simulink model "discretization_example_student"  (R2022b)
settings: Solver=ode4  StartTime=0.0  StopTime=timeEnd  FixedStep=timeStep  RelTol=1e-3
values from neighbouring files (symbols this model uses):
  stateInit = [1; 0.5]    [discretization_example_init.m]
  timeStep = 1e-3    (= 0.001)    [discretization_example_init.m]
undefined symbols (not defined in the file or in its folder): sys
settings Model: Creator=maam  LastModifiedBy=15043
settings SolverCC: AlgebraicLoopSolver=TrustRegion
settings DebuggingCC: UnconnectedInputMsg=warning  UnconnectedOutputMsg=warning  UnconnectedLineMsg=warning  SFMachineParentedDataDiag=warning  ArithmeticOperatorsInVariantConditions=warning
settings ModelReferenceCC: EnableRefExpFcnMdlSchedulingChecks=on
settings SFSimCC: CustomCodeUndefinedFunction=UseInterfaceOnly
settings CodeAppCC: StateflowObjectComments=on

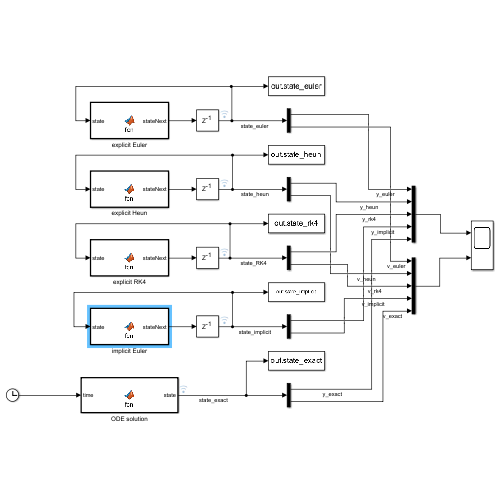
[thumbnail: Simulink's stored preview of the top-level diagram]
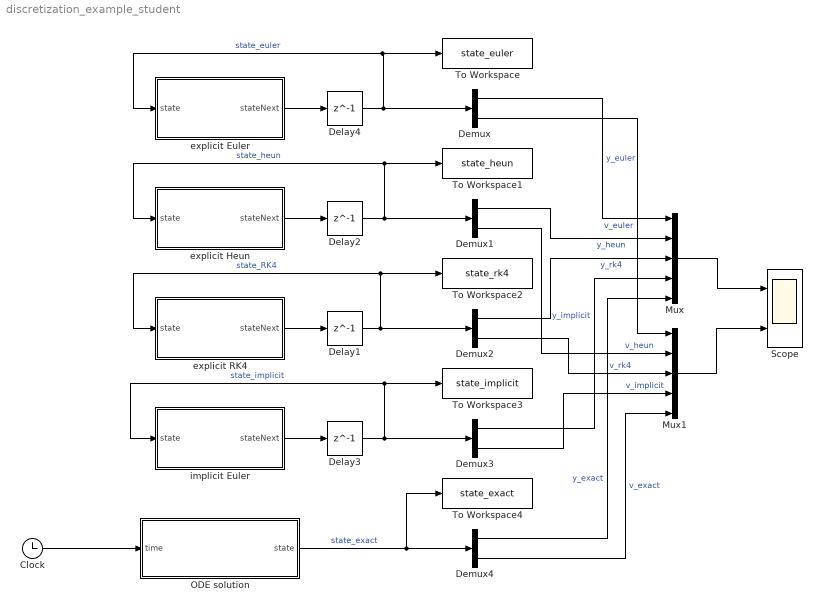
== system discretization_example_student ==
  Clock : Clock
  Delay{1..4} (4 alike) : Delay  DelayLength=1  InitialCondition=stateInit
  Demux{,1..4} (5 alike) : Demux  Outputs=2
  Mux : Mux  Inputs=5
  Mux1 : Mux  Inputs=5
  ODE solution : MATLAB Function  TreatAsAtomicUnit=on
  Scope : Scope  NumInputPorts=2
  To Workspace : ToWorkspace  VariableName=state_euler  SaveFormat=Timeseries  SampleTime=-1
  To Workspace1 : ToWorkspace  VariableName=state_heun  SaveFormat=Timeseries  SampleTime=-1
  To Workspace2 : ToWorkspace  VariableName=state_rk4  SaveFormat=Timeseries  SampleTime=-1
  To Workspace3 : ToWorkspace  VariableName=state_implicit  SaveFormat=Timeseries  SampleTime=-1
  To Workspace4 : ToWorkspace  VariableName=state_exact  SaveFormat=Timeseries  SampleTime=-1
  explicit Euler : MATLAB Function  TreatAsAtomicUnit=on
  explicit Heun : MATLAB Function  TreatAsAtomicUnit=on
  explicit RK4 : MATLAB Function  TreatAsAtomicUnit=on
  implicit Euler : MATLAB Function  TreatAsAtomicUnit=on
  wires:
  explicit Euler/1(stateNext) -> Delay4/1
  implicit Euler/1(stateNext) -> Delay3/1
  Clock/1 -> ODE solution/1(time)
  ODE solution/1(state) -> Demux4/1, To Workspace4/1  "state_exact"
  explicit RK4/1(stateNext) -> Delay1/1
  explicit Heun/1(stateNext) -> Delay2/1
  Delay3/1 -> Demux3/1, implicit Euler/1(state), To Workspace3/1  "state_implicit"
  Delay1/1 -> Demux2/1, To Workspace2/1, explicit RK4/1(state)  "state_RK4"
  Delay2/1 -> Demux1/1, To Workspace1/1, explicit Heun/1(state)  "state_heun"
  Delay4/1 -> Demux/1, To Workspace/1, explicit Euler/1(state)  "state_euler"
  Mux1/1 -> Scope/2
  Mux/1 -> Scope/1
  Demux/1 -> Mux/1  "y_euler"
  Demux/2 -> Mux1/1  "v_euler"
  Demux1/1 -> Mux/2  "y_heun"
  Demux2/1 -> Mux/3  "y_rk4"
  Demux3/1 -> Mux/4  "y_implicit"
  Demux4/1 -> Mux/5  "y_exact"
  Demux1/2 -> Mux1/2  "v_heun"
  Demux2/2 -> Mux1/3  "v_rk4"
  Demux3/2 -> Mux1/4  "v_implicit"
  Demux4/2 -> Mux1/5  "v_exact"

== matlab function discretization_example_student/explicit Heun ==
  data: state input size=2; stateNext output size=2; timeStep parameter; sys parameter
function stateNext = fcn(state, timeStep, sys)

    h = timeStep;
    f = mass_spring_model_ode(0,state,sys);

    yNext = state + h * f;
    stateNext = state + h/2 * (f + mass_spring_model_ode(0+h,yNext,sys));


    function dy = mass_spring_model_ode(t, y, sys)
        % y(1) = p; y(2) = p_dot
        dy = zeros(2,1);
        dy(1) = y(2); 
        dy(2) = (-1/sys.mass)*(sys.damping*y(2) + sys.stiffness*y(1));
    end
end

== matlab function discretization_example_student/explicit Euler ==
  data: state input size=2; stateNext output size=2; timeStep parameter; sys parameter
function stateNext = fcn(state, timeStep, sys)

    h = timeStep;
    f = mass_spring_model_ode(0,state,sys);
    stateNext = state + h * f;
    
    function dy = mass_spring_model_ode(t, y, sys)
        % y(1) = p; y(2) = p_dot
        dy = zeros(2,1);
        dy(1) = y(2); 
        dy(2) = (-1/sys.mass)*(sys.damping*y(2) + sys.stiffness*y(1));
    end
end

== matlab function discretization_example_student/explicit RK4 ==
  data: state input size=2; stateNext output size=2; timeStep parameter; sys parameter
function stateNext = fcn(state, timeStep, sys)

    h = timeStep;
    s1 = mass_spring_model_ode(0,state,sys);
    s2 = mass_spring_model_ode(0+h/2,state+h/2*s1,sys);
    s3 = mass_spring_model_ode(0+h/2,state+h/2*s2,sys);
    s4 = mass_spring_model_ode(0+h,state+h*s3,sys);


    stateNext = state + h/6 * (s1+2*s2+2*s3+s4);

    function dy = mass_spring_model_ode(t, y, sys)
        % y(1) = p; y(2) = p_dot
        dy = zeros(2,1);
        dy(1) = y(2); 
        dy(2) = (-1/sys.mass)*(sys.damping*y(2) + sys.stiffness*y(1));
    end
end

== matlab function discretization_example_student/ODE solution ==
  data: time input; state output; stateInit parameter; sys parameter
function state = fcn(time, stateInit, sys)
    w_0 = sqrt(sys.stiffness/sys.mass);
    deta = sys.damping/(2*sys.mass);
    w = sqrt(w_0^2-deta^2);
    p0 = stateInit(1);
    p0_dot = stateInit(2);
    
    state = zeros(2,1);
    state(1) = exp(-deta*time)*(p0*cos(w*time)+(p0_dot + deta*p0)/w*sin(w*time));
    state(2) = exp(-deta*time)*( -p0*sin(w*time)*w + (p0_dot + deta*p0)*cos(w*time) ) - deta*state(1);
end

== matlab function discretization_example_student/implicit Euler ==
  data: state input size=2; stateNext output size=2; timeStep parameter; sys parameter
function stateNext = fcn(state, timeStep, sys)
    
    h = timeStep;
    Df = [0 1; -sys.stiffness/sys.mass -sys.damping/sys.mass];
    
    x0 = state;
    f = mass_spring_model_ode(0,x0,sys);
%     x1 = x0 - inv(eye(length(state))-h*Df)*(h*f);
% 
%     while (norm(x1-x0)>0.0001)
%         x0 = x1;
%         x1 = x0 - inv(eye(length(state))-h*Df)*(x0 - h*f - state);
%     end
% 
%     stateNext = x1;

    stateNext = (eye(length(state))-h*Df)\state;
    

    function dy = mass_spring_model_ode(t, y, sys)
        % y(1) = p; y(2) = p_dot
        dy = zeros(2,1);
        dy(1) = y(2); 
        dy(2) = (-1/sys.mass)*(sys.damping*y(2) + sys.stiffness*y(1));
    end
end
